simulink subsystem "Beta_Controller"  (R2023b)
settings: Solver=VariableStepAuto  StartTime=0.0  StopTime=10.0  RelTol=1e-3
settings Model: Creator=cyber  LastModifiedBy=cyber

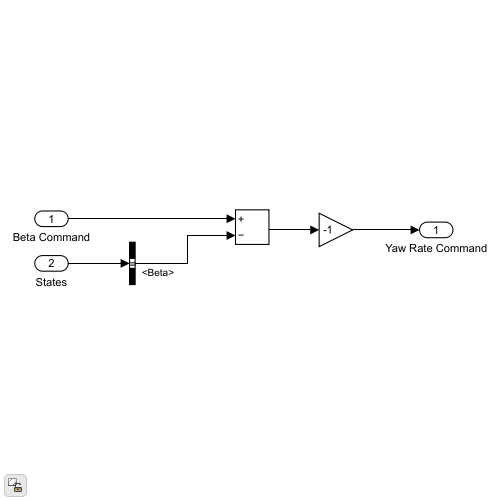
[thumbnail: Simulink's stored preview of the top-level diagram]
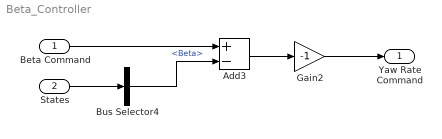
== system Beta_Controller ==
  Beta Command : Inport
  States : Inport  Port=2
  Add3 : Sum  Inputs=+-
  Bus Selector4 : BusSelector  OutputSignals=Beta
  Gain2 : Gain  Gain=-1
  Yaw Rate Command : Outport
  wires:
  Bus Selector4/1 -> Add3/2  "<Beta>"
  Beta Command/1 -> Add3/1
  Add3/1 -> Gain2/1
  States/1 -> Bus Selector4/1
  Gain2/1 -> Yaw Rate Command/1
